simulink model "M43"  (R2021b)
settings: Solver=VariableStepAuto  StartTime=0.0  StopTime=10.0  RelTol=1e-3
settings Model: Creator=abdul  LastModifiedBy=abdul

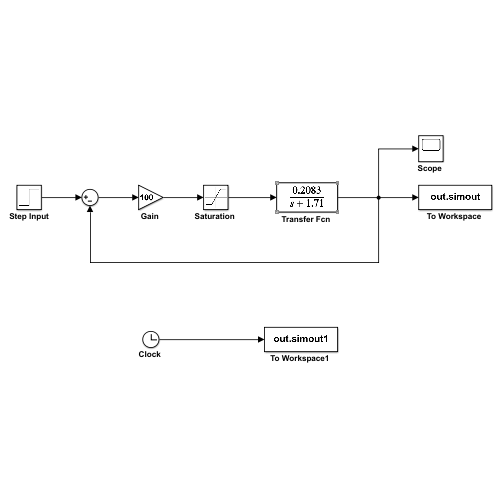
[thumbnail: Simulink's stored preview of the top-level diagram]
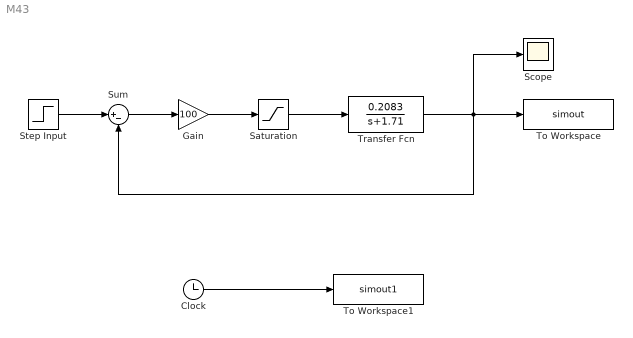
== system M43 ==
  "Clock " : Clock
  "Gain " : Gain  Gain=100
  "Saturation " : Saturate
  "Scope " : Scope
  Step Input : Step  Time=0  After=10  SampleTime=0
  Sum : Sum  Inputs=|+-
  "To Workspace " : ToWorkspace  VariableName=simout  SaveFormat=Timeseries  SampleTime=-1
  "To Workspace1 " : ToWorkspace  VariableName=simout1  SaveFormat=Timeseries  SampleTime=-1
  "Transfer Fcn " : TransferFcn  Numerator=[0.2083]  Denominator=[1 1.71]
  wires:
  "Clock "/1 -> "To Workspace1 "/1
  "Gain "/1 -> "Saturation "/1
  Sum/1 -> "Gain "/1
  Step Input/1 -> Sum/1
  "Saturation "/1 -> "Transfer Fcn "/1
  "Transfer Fcn "/1 -> Sum/2, "Scope "/1, "To Workspace "/1
